simulink library "MSP_FSW_lib"  (R2016b)
settings: Solver=VariableStepAuto  StartTime=0.0  StopTime=10.0  RelTol=1e-3
undefined symbols (not defined in the file): cmd_MT_fsw_dv, fsw_params, sc_mode
libraries: CAN_out_lib x1, extended_kalman_filter_lib x1, actuator_processing x1, bus_stubs_fsw x1, command_generation x1, env_estimation_lib x1, mode_selection x1, target_generation_lib x1
settings Model: Creator=taylorreynolds  LastModifiedBy=Taylor

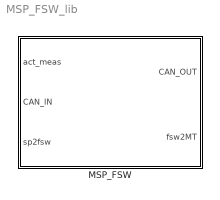
== system MSP_FSW_lib ==
  MSP_FSW : Subsystem

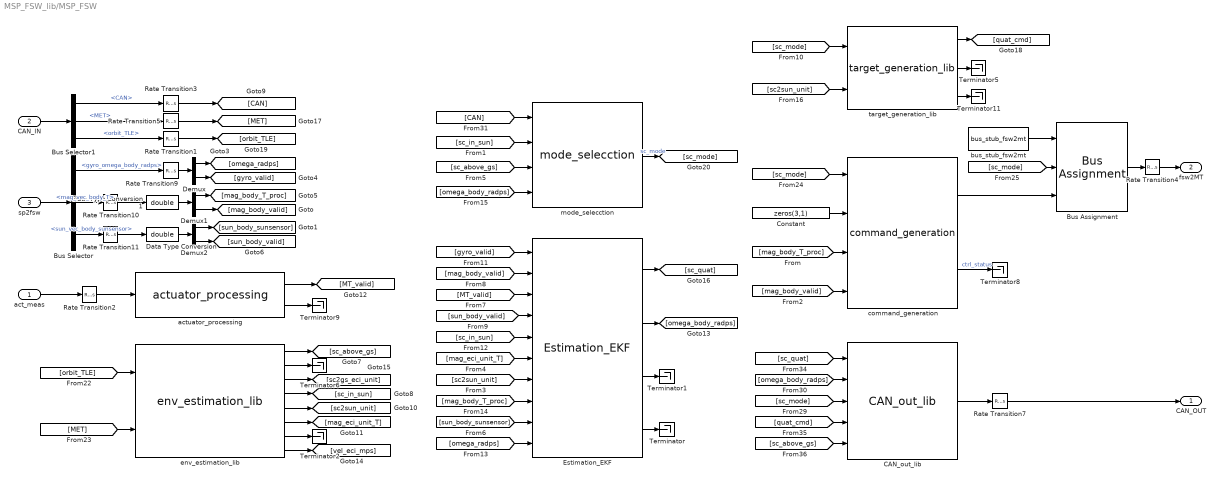
== system MSP_FSW_lib/MSP_FSW ==
  act_meas : Inport
  CAN_IN : Inport  Port=2  OutDataTypeStr=Bus: CAN_IN
  sp2fsw : Inport  Port=3  OutDataTypeStr=Bus: sp2fsw
  Bus Assignment : BusAssignment  AssignedSignals=sc_mode,cmd_MT_fsw_dv
  Bus Selector : BusSelector  OutputSignals=gyro_omega_body_radps,mag_vec_body_T,sun_vec_body_sunsensor
  Bus Selector1 : BusSelector  OutputSignals=CAN,MET,orbit_TLE
  CAN_out_lib : CAN_out_lib/CAN_out_lib
  Constant : Constant  Value=zeros(3,1)
  Data Type Conversion : DataTypeConversion  OutDataTypeStr=double
  Data Type Conversion1 : DataTypeConversion  OutDataTypeStr=double
  Demux : Demux  Outputs=[3 1]
  Demux1 : Demux  Outputs=[3 1]
  Demux2 : Demux  Outputs=[3 1]
  "Estimation_EKF " : extended_kalman_filter_lib/Estimation_EKF 
  Rate Transition1 : RateTransition  X0=fsw_params.bus.orbit_tle  OutPortSampleTime=fsw_params.sample_time_s
  Rate Transition{2,9..11} (4 alike) : RateTransition  OutPortSampleTime=fsw_params.sample_time_s
  Rate Transition3 : RateTransition  X0=fsw_params.bus.CAN_ic  OutPortSampleTime=fsw_params.sample_time_s
  Rate Transition4 : RateTransition
  Rate Transition5 : RateTransition  X0=fsw_params.bus.MET_epoch  OutPortSampleTime=fsw_params.sample_time_s
  Rate Transition7 : RateTransition
  Terminator{,1..2,5..6,8..9,11} (8 alike) : Terminator
  actuator_processing : actuator_processing/actuator_processing
  bus_stub_fsw2mt : bus_stubs_fsw/bus_stub_fsw2mt
  command_generation : command_generation/command_generation
  env_estimation_lib : env_estimation_lib/env_estimation_lib
  mode_selecction : mode_selection/mode_selecction
  target_generation_lib : target_generation_lib/target_generation_lib
  CAN_OUT : Outport
  fsw2MT : Outport  Port=2
  wires:
  Rate Transition3/1 -> [CAN]
  Bus Selector1/1 -> Rate Transition3/1  "<CAN>"
  Rate Transition11/1 -> Data Type Conversion/1
  Rate Transition9/1 -> Demux/1
  [sc_above_gs] -> mode_selecction/3
  env_estimation_lib/1 -> [sc_above_gs]
  "Estimation_EKF "/1 -> [sc_quat]
  command_generation/2 -> Terminator8/1  "ctrl_status"
  [mag_body_valid] -> command_generation/4
  [sc2sun_unit] -> "Estimation_EKF "/7
  [mag_eci_unit_T] -> "Estimation_EKF "/6
  [mag_body_T_proc] -> "Estimation_EKF "/8
  [sun_body_sunsensor] -> "Estimation_EKF "/9
  [omega_radps] -> "Estimation_EKF "/10
  env_estimation_lib/3 -> [sc2gs_eci_unit]
  env_estimation_lib/2 -> Terminator6/1
  env_estimation_lib/8 -> [vel_eci_mps]
  env_estimation_lib/7 -> Terminator2/1
  env_estimation_lib/6 -> [mag_eci_unit_T]
  env_estimation_lib/5 -> [sc2sun_unit]
  "Estimation_EKF "/3 -> Terminator1/1
  "Estimation_EKF "/4 -> Terminator/1
  [sc_in_sun] -> "Estimation_EKF "/5
  [sun_body_valid] -> "Estimation_EKF "/4
  [MT_valid] -> "Estimation_EKF "/3
  env_estimation_lib/4 -> [sc_in_sun]
  [gyro_valid] -> "Estimation_EKF "/1
  [mag_body_valid] -> "Estimation_EKF "/2
  [sc_in_sun] -> mode_selecction/2
  Bus Selector/1 -> Rate Transition9/1  "<gyro_omega_body_radps>"
  Demux/1 -> [omega_radps]
  Demux/2 -> [gyro_valid]
  Bus Selector/2 -> Rate Transition10/1  "<mag_vec_body_T>"
  Rate Transition10/1 -> Data Type Conversion1/1
  Bus Selector/3 -> Rate Transition11/1  "<sun_vec_body_sunsensor>"
  Demux2/1 -> [sun_body_sunsensor]
  Demux2/2 -> [sun_body_valid]
  act_meas/1 -> Rate Transition2/1
  actuator_processing/1 -> [MT_valid]
  actuator_processing/2 -> Terminator9/1
  "Estimation_EKF "/2 -> [omega_body_radps]
  [omega_body_radps] -> mode_selecction/4
  [sc2sun_unit] -> target_generation_lib/2
  target_generation_lib/1 -> [quat_cmd]
  target_generation_lib/2 -> Terminator5/1
  bus_stub_fsw2mt/1 -> Bus Assignment/1
  Bus Assignment/1 -> Rate Transition4/1
  CAN_out_lib/1 -> Rate Transition7/1
  sp2fsw/1 -> Bus Selector/1
  Rate Transition2/1 -> actuator_processing/1
  CAN_IN/1 -> Bus Selector1/1
  Rate Transition4/1 -> fsw2MT/1
  Rate Transition7/1 -> CAN_OUT/1
  [CAN] -> mode_selecction/1
  [sc_mode] -> CAN_out_lib/3
  [omega_body_radps] -> CAN_out_lib/2
  [sc_quat] -> CAN_out_lib/1
  [sc_above_gs] -> CAN_out_lib/5
  target_generation_lib/3 -> Terminator11/1
  [quat_cmd] -> CAN_out_lib/4
  [mag_body_T_proc] -> command_generation/3
  command_generation/1 -> Bus Assignment/3
  Constant/1 -> command_generation/2
  Rate Transition1/1 -> [orbit_TLE]
  Bus Selector1/3 -> Rate Transition1/1  "<orbit_TLE>"
  [orbit_TLE] -> env_estimation_lib/1
  [MET] -> env_estimation_lib/2
  mode_selecction/1 -> [sc_mode]  "sc_mode"
  [sc_mode] -> target_generation_lib/1
  [sc_mode] -> command_generation/1
  [sc_mode] -> Bus Assignment/2
  Rate Transition5/1 -> [MET]
  Bus Selector1/2 -> Rate Transition5/1  "<MET>"
  Demux1/1 -> [mag_body_T_proc]
  Demux1/2 -> [mag_body_valid]
  Data Type Conversion/1 -> Demux2/1
  Data Type Conversion1/1 -> Demux1/1
